simulink model "model2"  (R2018b)
settings: Solver=VariableStepAuto  StartTime=1.0  StopTime=10.0  RelTol=1e-3
settings Model: Creator=LimeTheCoder  LastModifiedBy=LimeTheCoder

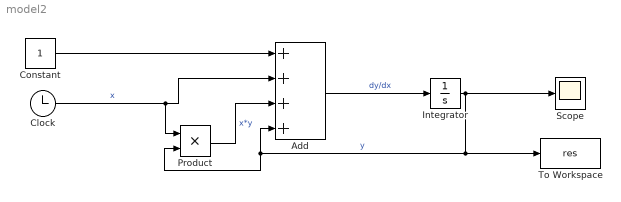
== system model2 ==
  Add : Sum  Inputs=++++
  Clock : Clock
  Constant : Constant
  Integrator : Integrator  InitialCondition=7
  Product : Product
  Scope : Scope
  To Workspace : ToWorkspace  VariableName=res  SampleTime=-1
      settings: Save2DSignal=2-D array (concatenate along first dimension)
  wires:
  Clock/1 -> Product/1, Add/2  "x"
  Constant/1 -> Add/1
  Add/1 -> Integrator/1  "dy/dx"
  Integrator/1 -> To Workspace/1, Product/2, Add/4, Scope/1  "y"
  Product/1 -> Add/3  "x*y"
